simulink model "motor_faulty"  (Simulink 10.1)
settings: Solver=ode45  StartTime=0.0  StopTime=m_time  MaxStep=0.001  RelTol=1e-3  EnableMultiTasking=on
values from neighbouring files (symbols this model uses):
  ACR_d = mf_PI_c2d(ACR_c)    [ini_faulty.m]    (also in ini_normal.m)
  alpha = 0.006666666666    [ini_faulty.m]    (also in ini_normal.m)
  ASR_d = mf_PI_c2d(ASR_c)    [ini_faulty.m]    (also in ini_normal.m)
  beta = 0.125    [ini_faulty.m]    (also in ini_normal.m)
  Ce = 0.133    [ini_faulty.m]    (also in ini_normal.m)
  Ks = 36    [ini_faulty.m]    (also in ini_normal.m)
  m_load10e_final = -m_load    (= 0)    [ini_faulty.m]    (also in ini_normal.m)
  m_load10e_ini = 0    [ini_faulty.m]    (also in ini_normal.m)
  m_load10e_steptime = m_load10s_steptime+m_steeltime    (= 58)    [ini_faulty.m]    (also in ini_normal.m)
  m_load10s_final = m_load    (= 0)    [ini_faulty.m]    (also in ini_normal.m)
  m_load10s_ini = 0    [ini_faulty.m]    (also in ini_normal.m)
  m_load10s_steptime = m_load9e_steptime+m_idletime    (= 55)    [ini_faulty.m]    (also in ini_normal.m)
  m_load11e_final = -m_load    (= 0)    [ini_faulty.m]    (also in ini_normal.m)
  m_load11e_ini = 0    [ini_faulty.m]    (also in ini_normal.m)
  m_load11e_steptime = m_load11s_steptime+m_steeltime    (= 63)    [ini_faulty.m]    (also in ini_normal.m)
  m_load11s_final = m_load    (= 0)    [ini_faulty.m]    (also in ini_normal.m)
  m_load11s_ini = 0    [ini_faulty.m]    (also in ini_normal.m)
  m_load11s_steptime = m_load10e_steptime+m_idletime    (= 60)    [ini_faulty.m]    (also in ini_normal.m)
  m_load1e_final = -m_load    (= 0)    [ini_faulty.m]    (also in ini_normal.m)
  m_load1e_ini = 0    [ini_faulty.m]    (also in ini_normal.m)
  m_load1e_steptime = m_load1s_steptime+m_steeltime    (= 13)    [ini_faulty.m]    (also in ini_normal.m)
  m_load1s_final = m_load    (= 0)    [ini_faulty.m]    (also in ini_normal.m)
  m_load1s_ini = 0    [ini_faulty.m]    (also in ini_normal.m)
  m_load1s_steptime = 10    [ini_faulty.m]    (also in ini_normal.m)
  m_load2e_final = -m_load    (= 0)    [ini_faulty.m]    (also in ini_normal.m)
  m_load2e_ini = 0    [ini_faulty.m]    (also in ini_normal.m)
  m_load2e_steptime = m_load2s_steptime+m_steeltime    (= 18)    [ini_faulty.m]    (also in ini_normal.m)
  m_load2s_final = m_load    (= 0)    [ini_faulty.m]    (also in ini_normal.m)
  m_load2s_ini = 0    [ini_faulty.m]    (also in ini_normal.m)
  m_load2s_steptime = m_load1e_steptime+m_idletime    (= 15)    [ini_faulty.m]    (also in ini_normal.m)
  m_load3e_final = -m_load    (= 0)    [ini_faulty.m]    (also in ini_normal.m)
  m_load3e_ini = 0    [ini_faulty.m]    (also in ini_normal.m)
  m_load3e_steptime = m_load3s_steptime+m_steeltime    (= 23)    [ini_faulty.m]    (also in ini_normal.m)
  m_load3s_final = m_load    (= 0)    [ini_faulty.m]    (also in ini_normal.m)
  m_load3s_ini = 0    [ini_faulty.m]    (also in ini_normal.m)
  m_load3s_steptime = m_load2e_steptime+m_idletime    (= 20)    [ini_faulty.m]    (also in ini_normal.m)
  m_load4e_final = -m_load    (= 0)    [ini_faulty.m]    (also in ini_normal.m)
  m_load4e_ini = 0    [ini_faulty.m]    (also in ini_normal.m)
  m_load4e_steptime = m_load4s_steptime+m_steeltime    (= 28)    [ini_faulty.m]    (also in ini_normal.m)
  m_load4s_final = m_load    (= 0)    [ini_faulty.m]    (also in ini_normal.m)
  m_load4s_ini = 0    [ini_faulty.m]    (also in ini_normal.m)
  m_load4s_steptime = m_load3e_steptime+m_idletime    (= 25)    [ini_faulty.m]    (also in ini_normal.m)
  m_load5e_final = -m_load    (= 0)    [ini_faulty.m]    (also in ini_normal.m)
  m_load5e_ini = 0    [ini_faulty.m]    (also in ini_normal.m)
  m_load5e_steptime = m_load5s_steptime+m_steeltime    (= 33)    [ini_faulty.m]    (also in ini_normal.m)
  m_load5s_final = m_load    (= 0)    [ini_faulty.m]    (also in ini_normal.m)
  m_load5s_ini = 0    [ini_faulty.m]    (also in ini_normal.m)
  m_load5s_steptime = m_load4e_steptime+m_idletime    (= 30)    [ini_faulty.m]    (also in ini_normal.m)
  m_load6e_final = -m_load    (= 0)    [ini_faulty.m]    (also in ini_normal.m)
  m_load6e_ini = 0    [ini_faulty.m]    (also in ini_normal.m)
  m_load6e_steptime = m_load6s_steptime+m_steeltime    (= 38)    [ini_faulty.m]    (also in ini_normal.m)
  m_load6s_final = m_load    (= 0)    [ini_faulty.m]    (also in ini_normal.m)
  m_load6s_ini = 0    [ini_faulty.m]    (also in ini_normal.m)
  m_load6s_steptime = m_load5e_steptime+m_idletime    (= 35)    [ini_faulty.m]    (also in ini_normal.m)
  m_load7e_final = -m_load    (= 0)    [ini_faulty.m]    (also in ini_normal.m)
  m_load7e_ini = 0    [ini_faulty.m]    (also in ini_normal.m)
  m_load7e_steptime = m_load7s_steptime+m_steeltime    (= 43)    [ini_faulty.m]    (also in ini_normal.m)
  m_load7s_final = m_load    (= 0)    [ini_faulty.m]    (also in ini_normal.m)
  m_load7s_ini = 0    [ini_faulty.m]    (also in ini_normal.m)
  m_load7s_steptime = m_load6e_steptime+m_idletime    (= 40)    [ini_faulty.m]    (also in ini_normal.m)
  m_load8e_final = -m_load    (= 0)    [ini_faulty.m]    (also in ini_normal.m)
  m_load8e_ini = 0    [ini_faulty.m]    (also in ini_normal.m)
  m_load8e_steptime = m_load8s_steptime+m_steeltime    (= 48)    [ini_faulty.m]    (also in ini_normal.m)
  m_load8s_final = m_load    (= 0)    [ini_faulty.m]    (also in ini_normal.m)
  m_load8s_ini = 0    [ini_faulty.m]    (also in ini_normal.m)
  m_load8s_steptime = m_load7e_steptime+m_idletime    (= 45)    [ini_faulty.m]    (also in ini_normal.m)
  m_load9e_final = -m_load    (= 0)    [ini_faulty.m]    (also in ini_normal.m)
  m_load9e_ini = 0    [ini_faulty.m]    (also in ini_normal.m)
  m_load9e_steptime = m_load9s_steptime+m_steeltime    (= 53)    [ini_faulty.m]    (also in ini_normal.m)
  m_load9s_final = m_load    (= 0)    [ini_faulty.m]    (also in ini_normal.m)
  m_load9s_ini = 0    [ini_faulty.m]    (also in ini_normal.m)
  m_load9s_steptime = m_load8e_steptime+m_idletime    (= 50)    [ini_faulty.m]    (also in ini_normal.m)
  m_ts = 0.01    [ini_faulty.m]    (also in ini_normal.m)
  n_mean1 = 0    [ini_faulty.m]    (also in ini_normal.m)
  n_mean2 = 0    [ini_faulty.m]    (also in ini_normal.m)
  n_seed1 = floor(1000*rand(1))    [ini_faulty.m]    (also in ini_normal.m)
  n_seed2 = floor(1000*rand(1))    [ini_faulty.m]    (also in ini_normal.m)
  n_var1 = 500    [ini_faulty.m]    (also in ini_normal.m)
  n_var2 = 100    [ini_faulty.m]    (also in ini_normal.m)
  R = 0.58    [ini_faulty.m]    (also in ini_normal.m)
  Ti = 0.0313    [ini_faulty.m]    (also in ini_normal.m)
  Tm = 0.063    [ini_faulty.m]    (also in ini_normal.m)
  Ts = 0.0017    [ini_faulty.m]    (also in ini_normal.m)
undefined symbols (not defined in the file or in its folder): sigbuilder_block
settings Model: Creator=Hao  LastModifiedBy=Administrator
settings DataIOCC: LimitDataPoints=on  SignalLoggingSaveFormat=ModelDataLogs
settings OptimizationCC: ExpressionDepthLimit=2147483647
settings DebuggingCC: SolverPrmCheckMsg=warning  FcnCallInpInsideContextMsg=warning  StateNameClashWarn=warning
settings ConfigComp: CovSFcnEnable=off

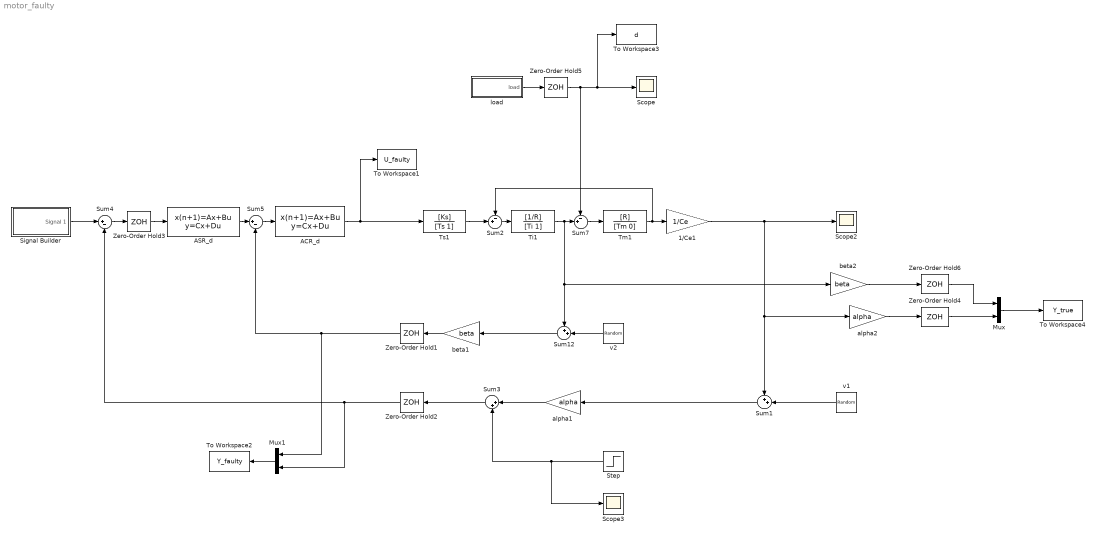
== system motor_faulty ==
  1/Ce1 : Gain  Gain=1/Ce
  ACR_d : DiscreteStateSpace  A=ACR_d.A  B=ACR_d.B  C=ACR_d.C  D=ACR_d.D  SampleTime=-1
  ASR_d : DiscreteStateSpace  A=ASR_d.A  B=ASR_d.B  C=ASR_d.C  D=ASR_d.D  SampleTime=-1
  Mux : Mux  Inputs=2
  Mux1 : Mux  Inputs=2
  Scope : Scope
  Scope2 : Scope
  Scope3 : Scope
  Signal Builder : Subsystem  Tag=STV Subsys  LoadFcn=sigbuilder_block('load');  StartFcn=sigbuilder_block('start');  StopFcn=sigbuilder_block('stop');  ClipboardFcn=sigbuilder_block('clipboard');  mask(Sigbuilder block){tuvar=[0:10]}
      mask help: Simulink:masks:SigbuilderBlock_MD
      mask init:
      | if ~strcmp(get_param(bdroot(gcbh),'SimulationStatus'),'stopped') tuvar = sigbuilder_block('maskInit'); end
      settings: CopyFcn=sigbuilder_block('copy');  DeleteFcn=sigbuilder_block('delete');  ModelCloseFcn=sigbuilder_block('modelClose');  PreSaveFcn=sigbuilder_block('preSave');  PauseFcn=sigbuilder_block('pause');  ContinueFcn=sigbuilder_block('continue');  NameChangeFcn=sigbuilder_block('namechange');  OpenFcn=sigbuilder_block('open',[5.5 0 949 449 ]);  CloseFcn=sigbuilder_block('close');
      mask Display: plot(0, 0, 100, 100,[2, 2, 32, 32, 2], [68, 8, 8, 68, 68],[32, 2], [38, 38], [32, 19, 2],[53, 60, 44], [32, 17, 17, 2],[16, 16, 31, 31]);txt = getActiveGroup(gcbh);text(2, 100, txt,'verticalAlignment', 'top');
  Step : Step  Time=8  SampleTime=m_ts
  Sum1 : Sum  Inputs=++|
  Sum12 : Sum  Inputs=++|
  Sum2 : Sum  Inputs=-+|
  Sum3 : Sum  Inputs=|++
  Sum4 : Sum  Inputs=|+-
  Sum5 : Sum  Inputs=|+-
  Sum7 : Sum  Inputs=-+|
  Ti1 : TransferFcn  Numerator=[1/R]  Denominator=[Ti 1]
  Tm1 : TransferFcn  Numerator=[R]  Denominator=[Tm 0]
  To Workspace1 : ToWorkspace  VariableName=U_faulty  SampleTime=-1
      settings: Save2DSignal=2-D array (concatenate along first dimension)
  To Workspace2 : ToWorkspace  VariableName=Y_faulty  SampleTime=-1
      settings: Save2DSignal=2-D array (concatenate along first dimension)
  To Workspace3 : ToWorkspace  VariableName=d  SampleTime=-1
      settings: Save2DSignal=2-D array (concatenate along first dimension)
  To Workspace4 : ToWorkspace  VariableName=Y_true  SampleTime=-1
      settings: Save2DSignal=2-D array (concatenate along first dimension)
  Ts1 : TransferFcn  Numerator=[Ks]  Denominator=[Ts 1]
  Zero-Order Hold{1..6} (6 alike) : ZeroOrderHold  SampleTime=m_ts
  alpha1 : Gain  Gain=alpha
  alpha2 : Gain  Gain=alpha
  beta1 : Gain  Gain=beta
  beta2 : Gain  Gain=beta
  load : Subsystem
  v1 : RandomNumber  Mean=n_mean1  Variance=n_var1  Seed=n_seed1  SampleTime=m_ts
  v2 : RandomNumber  Mean=n_mean2  Variance=n_var2  Seed=n_seed2  SampleTime=m_ts
  wires:
  Sum4/1 -> Zero-Order Hold3/1
  Sum5/1 -> ACR_d/1
  Ts1/1 -> Sum2/2
  Sum2/1 -> Ti1/1
  Ti1/1 -> beta2/1, Sum12/1, Sum7/2
  Tm1/1 -> 1/Ce1/1, Sum2/1
  Sum7/1 -> Tm1/1
  beta1/1 -> Zero-Order Hold1/1
  Zero-Order Hold1/1 -> Mux1/1, Sum5/2
  ACR_d/1 -> To Workspace1/1, Ts1/1
  v2/1 -> Sum12/2
  Sum12/1 -> beta1/1
  Zero-Order Hold2/1 -> Mux1/2, Sum4/2
  Zero-Order Hold5/1 -> Sum7/1, To Workspace3/1, Scope/1
  load/1(load) -> Zero-Order Hold5/1
  ASR_d/1 -> Sum5/1
  Zero-Order Hold3/1 -> ASR_d/1
  Signal Builder/1(Signal 1) -> Sum4/1
  Step/1 -> Sum3/2, Scope3/1
  alpha1/1 -> Sum3/1
  Sum3/1 -> Zero-Order Hold2/1
  Sum1/1 -> alpha1/1
  v1/1 -> Sum1/2
  alpha2/1 -> Zero-Order Hold4/1
  beta2/1 -> Zero-Order Hold6/1
  Mux/1 -> To Workspace4/1
  1/Ce1/1 -> Scope2/1, alpha2/1, Sum1/1
  Zero-Order Hold4/1 -> Mux/2
  Zero-Order Hold6/1 -> Mux/1
  Mux1/1 -> To Workspace2/1

== system motor_faulty/Signal Builder ==
  Demux : Demux  Tag=STV Demux  Outputs=1
      settings: DisplayOption=none
  FromWs : FromWorkspace  Tag=STV FromWs  VariableName=tuvar  SigBuilderData=DataTag0  VnvData=DataTag1
      SigBuilderData=|
      | common.afterFinalStr = 'Extrapolate'
      | common.sampleTime = 0
      | dataSet.timeRange = [0 10]
      | dataSet.name = 'Group 1'
      | sbobj.Groups.Name = 'Group 1'
      | sbobj.Groups.Signals.Name = 'Signal 1'
      | sbobj.Groups.Signals.XData = [0 4 4 6 6 10]
      | sbobj.Groups.Signals.YData = [5 5 8 8 10 10]
  Signal 1 : Outport  Tag=STV Outport
  wires:
  FromWs/1 -> Demux/1
  Demux/1 -> Signal 1/1

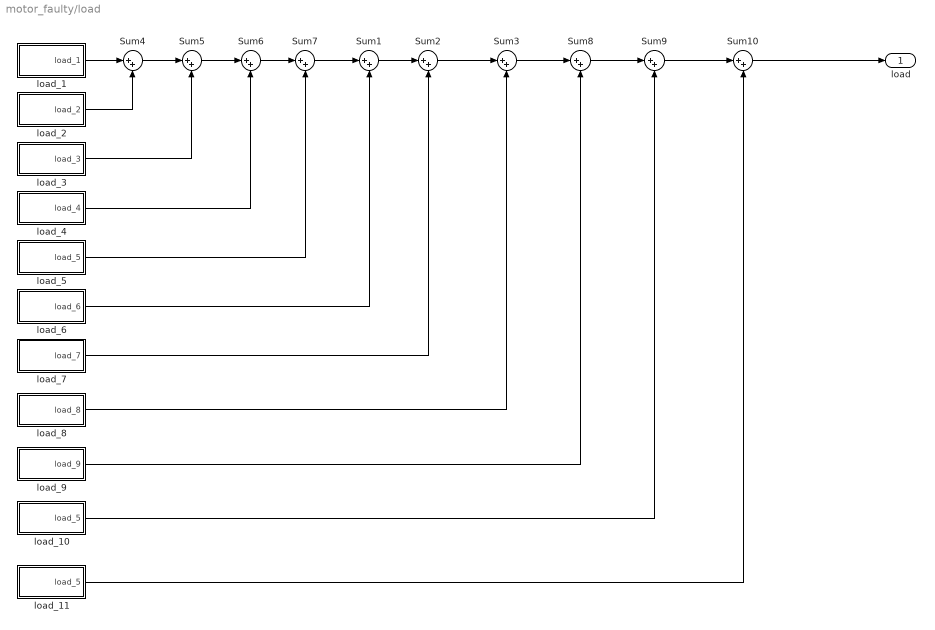
== system motor_faulty/load ==
  Sum{1..10} (10 alike) : Sum  Inputs=|++
  load_1 : Subsystem
  load_10 : Subsystem
  load_11 : Subsystem
  load_2 : Subsystem
  load_3 : Subsystem
  load_4 : Subsystem
  load_5 : Subsystem
  load_6 : Subsystem
  load_7 : Subsystem
  load_8 : Subsystem
  load_9 : Subsystem
  load : Outport
  wires:
  load_1/1(load_1) -> Sum4/1
  load_2/1(load_2) -> Sum4/2
  Sum4/1 -> Sum5/1
  load_3/1(load_3) -> Sum5/2
  Sum5/1 -> Sum6/1
  load_4/1(load_4) -> Sum6/2
  Sum6/1 -> Sum7/1
  load_5/1(load_5) -> Sum7/2
  load_6/1(load_6) -> Sum1/2
  load_7/1(load_7) -> Sum2/2
  load_8/1(load_8) -> Sum3/2
  load_9/1(load_9) -> Sum8/2
  load_10/1(load_5) -> Sum9/2
  Sum7/1 -> Sum1/1
  Sum1/1 -> Sum2/1
  Sum2/1 -> Sum3/1
  Sum3/1 -> Sum8/1
  Sum8/1 -> Sum9/1
  Sum9/1 -> Sum10/1
  load_11/1(load_5) -> Sum10/2
  Sum10/1 -> load/1

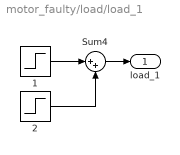
== system motor_faulty/load/load_1 ==
  1 : Step  Time=m_load1s_steptime  Before=m_load1s_ini  After=m_load1s_final  SampleTime=0
  2 : Step  Time=m_load1e_steptime  Before=m_load1e_ini  After=m_load1e_final  SampleTime=0
  Sum4 : Sum  Inputs=|++
  load_1 : Outport
  wires:
  1/1 -> Sum4/1
  2/1 -> Sum4/2
  Sum4/1 -> load_1/1

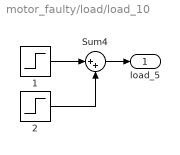
== system motor_faulty/load/load_10 ==
  1 : Step  Time=m_load10s_steptime  Before=m_load10s_ini  After=m_load10s_final  SampleTime=0
  2 : Step  Time=m_load10e_steptime  Before=m_load10e_ini  After=m_load10e_final  SampleTime=0
  Sum4 : Sum  Inputs=|++
  load_5 : Outport
  wires:
  1/1 -> Sum4/1
  2/1 -> Sum4/2
  Sum4/1 -> load_5/1

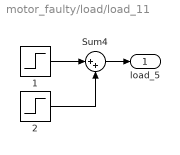
== system motor_faulty/load/load_11 ==
  1 : Step  Time=m_load11s_steptime  Before=m_load11s_ini  After=m_load11s_final  SampleTime=0
  2 : Step  Time=m_load11e_steptime  Before=m_load11e_ini  After=m_load11e_final  SampleTime=0
  Sum4 : Sum  Inputs=|++
  load_5 : Outport
  wires:
  Sum4/1 -> load_5/1
  2/1 -> Sum4/2
  1/1 -> Sum4/1

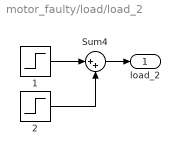
== system motor_faulty/load/load_2 ==
  1 : Step  Time=m_load2s_steptime  Before=m_load2s_ini  After=m_load2s_final  SampleTime=0
  2 : Step  Time=m_load2e_steptime  Before=m_load2e_ini  After=m_load2e_final  SampleTime=0
  Sum4 : Sum  Inputs=|++
  load_2 : Outport
  wires:
  Sum4/1 -> load_2/1
  2/1 -> Sum4/2
  1/1 -> Sum4/1

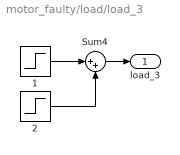
== system motor_faulty/load/load_3 ==
  1 : Step  Time=m_load3s_steptime  Before=m_load3s_ini  After=m_load3s_final  SampleTime=0
  2 : Step  Time=m_load3e_steptime  Before=m_load3e_ini  After=m_load3e_final  SampleTime=0
  Sum4 : Sum  Inputs=|++
  load_3 : Outport
  wires:
  1/1 -> Sum4/1
  2/1 -> Sum4/2
  Sum4/1 -> load_3/1

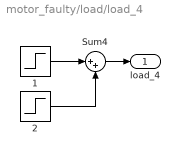
== system motor_faulty/load/load_4 ==
  1 : Step  Time=m_load4s_steptime  Before=m_load4s_ini  After=m_load4s_final  SampleTime=0
  2 : Step  Time=m_load4e_steptime  Before=m_load4e_ini  After=m_load4e_final  SampleTime=0
  Sum4 : Sum  Inputs=|++
  load_4 : Outport
  wires:
  Sum4/1 -> load_4/1
  2/1 -> Sum4/2
  1/1 -> Sum4/1

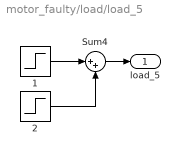
== system motor_faulty/load/load_5 ==
  1 : Step  Time=m_load5s_steptime  Before=m_load5s_ini  After=m_load5s_final  SampleTime=0
  2 : Step  Time=m_load5e_steptime  Before=m_load5e_ini  After=m_load5e_final  SampleTime=0
  Sum4 : Sum  Inputs=|++
  load_5 : Outport
  wires:
  1/1 -> Sum4/1
  2/1 -> Sum4/2
  Sum4/1 -> load_5/1

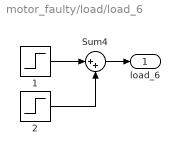
== system motor_faulty/load/load_6 ==
  1 : Step  Time=m_load6s_steptime  Before=m_load6s_ini  After=m_load6s_final  SampleTime=0
  2 : Step  Time=m_load6e_steptime  Before=m_load6e_ini  After=m_load6e_final  SampleTime=0
  Sum4 : Sum  Inputs=|++
  load_6 : Outport
  wires:
  1/1 -> Sum4/1
  2/1 -> Sum4/2
  Sum4/1 -> load_6/1

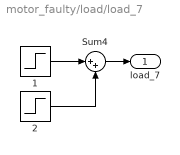
== system motor_faulty/load/load_7 ==
  1 : Step  Time=m_load7s_steptime  Before=m_load7s_ini  After=m_load7s_final  SampleTime=0
  2 : Step  Time=m_load7e_steptime  Before=m_load7e_ini  After=m_load7e_final  SampleTime=0
  Sum4 : Sum  Inputs=|++
  load_7 : Outport
  wires:
  1/1 -> Sum4/1
  2/1 -> Sum4/2
  Sum4/1 -> load_7/1

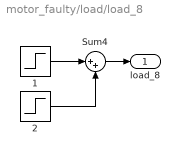
== system motor_faulty/load/load_8 ==
  1 : Step  Time=m_load8s_steptime  Before=m_load8s_ini  After=m_load8s_final  SampleTime=0
  2 : Step  Time=m_load8e_steptime  Before=m_load8e_ini  After=m_load8e_final  SampleTime=0
  Sum4 : Sum  Inputs=|++
  load_8 : Outport
  wires:
  1/1 -> Sum4/1
  2/1 -> Sum4/2
  Sum4/1 -> load_8/1

== system motor_faulty/load/load_9 ==
  1 : Step  Time=m_load9s_steptime  Before=m_load9s_ini  After=m_load9s_final  SampleTime=0
  2 : Step  Time=m_load9e_steptime  Before=m_load9e_ini  After=m_load9e_final  SampleTime=0
  Sum4 : Sum  Inputs=|++
  load_9 : Outport
  wires:
  1/1 -> Sum4/1
  2/1 -> Sum4/2
  Sum4/1 -> load_9/1
